simulink model "IEEE14_case"  (R2024b)
settings: Solver=FixedStepAuto  StartTime=0  StopTime=2  FixedStep=1e-7  RelTol=1e-3
values from neighbouring files (symbols this model uses):
  GFL_15_Bva = 0.009    [IEEE14_parameters.m]
  GFL_15_C_bus_pu = 7.179419    [IEEE14_parameters.m]
  GFL_15_f0 = 60    [IEEE14_parameters.m]
  GFL_15_I_id = 691.26967    [IEEE14_parameters.m]
  GFL_15_I_iq = 691.26967    [IEEE14_parameters.m]
  GFL_15_I_od = 45.2207    [IEEE14_parameters.m]
  GFL_15_I_oq = 45.2207    [IEEE14_parameters.m]
  GFL_15_I_pll = 0.78    [IEEE14_parameters.m]
  GFL_15_Kdi = 0.09    [IEEE14_parameters.m]
  GFL_15_Kdo = 0.9    [IEEE14_parameters.m]
  GFL_15_Kqi = 0.09    [IEEE14_parameters.m]
  GFL_15_Kqo = 0.9    [IEEE14_parameters.m]
  GFL_15_Lg_pu = 0.631447    [IEEE14_parameters.m]
  GFL_15_mode = 1    [IEEE14_parameters.m]
  GFL_15_P_id = 3.7166    [IEEE14_parameters.m]
  GFL_15_P_iq = 3.7166    [IEEE14_parameters.m]
  GFL_15_P_od = 0.4798    [IEEE14_parameters.m]
  GFL_15_P_oq = 0.4798    [IEEE14_parameters.m]
  GFL_15_P_pll = 290.42    [IEEE14_parameters.m]
  GFL_15_Qe_ref = 0.2    [IEEE14_parameters.m]
  GFL_15_Rg_pu = 0.024016    [IEEE14_parameters.m]
  GFL_15_Sbase = 1.000000e+4    (= 10000)    [IEEE14_parameters.m]
  GFL_15_Tdi = 0.01    [IEEE14_parameters.m]
  GFL_15_Tdo = 0.2    [IEEE14_parameters.m]
  GFL_15_Tqi = 0.01    [IEEE14_parameters.m]
  GFL_15_Tqo = 0.2    [IEEE14_parameters.m]
  GFL_15_Vbase = 380    [IEEE14_parameters.m]
  GFL_15_Vdc_ref = 1.011475    [IEEE14_parameters.m]
  GFL_15_Vdcbase = 700    [IEEE14_parameters.m]
  GFL_15_vq_ref = 0    [IEEE14_parameters.m]
  GFL_16_Bva = 0.002    [IEEE14_parameters.m]
  GFL_16_C_bus_pu = 7.179419    [IEEE14_parameters.m]
  GFL_16_f0 = 60    [IEEE14_parameters.m]
  GFL_16_I_id = 691.26967    [IEEE14_parameters.m]
  GFL_16_I_iq = 691.26967    [IEEE14_parameters.m]
  GFL_16_I_od = 45.2207    [IEEE14_parameters.m]
  GFL_16_I_oq = 45.2207    [IEEE14_parameters.m]
  GFL_16_I_pll = 0.78    [IEEE14_parameters.m]
  GFL_16_Kdi = 0.05    [IEEE14_parameters.m]
  GFL_16_Kdo = 0.5    [IEEE14_parameters.m]
  GFL_16_Kqi = 0.05    [IEEE14_parameters.m]
  GFL_16_Kqo = 0.5    [IEEE14_parameters.m]
  GFL_16_Lg_pu = 0.631447    [IEEE14_parameters.m]
  GFL_16_mode = 1    [IEEE14_parameters.m]
  GFL_16_P_id = 3.7166    [IEEE14_parameters.m]
  GFL_16_P_iq = 3.7166    [IEEE14_parameters.m]
  GFL_16_P_od = 0.4798    [IEEE14_parameters.m]
  GFL_16_P_oq = 0.4798    [IEEE14_parameters.m]
  GFL_16_P_pll = 290.42    [IEEE14_parameters.m]
  GFL_16_Qe_ref = 0.2    [IEEE14_parameters.m]
  GFL_16_Rg_pu = 0.024016    [IEEE14_parameters.m]
  GFL_16_Sbase = 1.000000e+4    (= 10000)    [IEEE14_parameters.m]
  GFL_16_Tdi = 0.01    [IEEE14_parameters.m]
  GFL_16_Tdo = 0.2    [IEEE14_parameters.m]
  GFL_16_Tqi = 0.01    [IEEE14_parameters.m]
  GFL_16_Tqo = 0.2    [IEEE14_parameters.m]
  GFL_16_Vbase = 380    [IEEE14_parameters.m]
  GFL_16_Vdc_ref = 1.01144    [IEEE14_parameters.m]
  GFL_16_Vdcbase = 700    [IEEE14_parameters.m]
  GFL_16_vq_ref = 0    [IEEE14_parameters.m]
  GFL_17_Bva = 0.002    [IEEE14_parameters.m]
  GFL_17_C_bus_pu = 7.179419    [IEEE14_parameters.m]
  GFL_17_f0 = 60    [IEEE14_parameters.m]
  GFL_17_I_id = 691.26967    [IEEE14_parameters.m]
  GFL_17_I_iq = 691.26967    [IEEE14_parameters.m]
  GFL_17_I_od = 45.2207    [IEEE14_parameters.m]
  GFL_17_I_oq = 45.2207    [IEEE14_parameters.m]
  GFL_17_I_pll = 0.78    [IEEE14_parameters.m]
  GFL_17_Kdi = 0.05    [IEEE14_parameters.m]
  GFL_17_Kdo = 0.5    [IEEE14_parameters.m]
  GFL_17_Kqi = 0.05    [IEEE14_parameters.m]
  GFL_17_Kqo = 0.5    [IEEE14_parameters.m]
  GFL_17_Lg_pu = 0.631447    [IEEE14_parameters.m]
  GFL_17_mode = 1    [IEEE14_parameters.m]
  GFL_17_P_id = 3.7166    [IEEE14_parameters.m]
  GFL_17_P_iq = 3.7166    [IEEE14_parameters.m]
  GFL_17_P_od = 0.4798    [IEEE14_parameters.m]
  GFL_17_P_oq = 0.4798    [IEEE14_parameters.m]
  GFL_17_P_pll = 290.42    [IEEE14_parameters.m]
  GFL_17_Qe_ref = 0.2    [IEEE14_parameters.m]
  GFL_17_Rg_pu = 0.024016    [IEEE14_parameters.m]
  GFL_17_Sbase = 1.000000e+4    (= 10000)    [IEEE14_parameters.m]
  GFL_17_Tdi = 0.01    [IEEE14_parameters.m]
  GFL_17_Tdo = 0.2    [IEEE14_parameters.m]
  GFL_17_Tqi = 0.01    [IEEE14_parameters.m]
  GFL_17_Tqo = 0.2    [IEEE14_parameters.m]
  GFL_17_Vbase = 380    [IEEE14_parameters.m]
  GFL_17_Vdc_ref = 1.011632    [IEEE14_parameters.m]
  GFL_17_Vdcbase = 700    [IEEE14_parameters.m]
  GFL_17_vq_ref = 0    [IEEE14_parameters.m]
  GFL_18_Bva = 0.002    [IEEE14_parameters.m]
  GFL_18_C_bus_pu = 7.179419    [IEEE14_parameters.m]
  GFL_18_f0 = 60    [IEEE14_parameters.m]
  GFL_18_I_id = 691.26967    [IEEE14_parameters.m]
  GFL_18_I_iq = 691.26967    [IEEE14_parameters.m]
  GFL_18_I_od = 45.2207    [IEEE14_parameters.m]
  GFL_18_I_oq = 45.2207    [IEEE14_parameters.m]
  GFL_18_I_pll = 0.78    [IEEE14_parameters.m]
  GFL_18_Kdi = 0.05    [IEEE14_parameters.m]
  GFL_18_Kdo = 0.5    [IEEE14_parameters.m]
  GFL_18_Kqi = 0.05    [IEEE14_parameters.m]
  GFL_18_Kqo = 0.5    [IEEE14_parameters.m]
  GFL_18_Lg_pu = 0.631447    [IEEE14_parameters.m]
  GFL_18_mode = 1    [IEEE14_parameters.m]
  GFL_18_P_id = 3.7166    [IEEE14_parameters.m]
  GFL_18_P_iq = 3.7166    [IEEE14_parameters.m]
  GFL_18_P_od = 0.4798    [IEEE14_parameters.m]
  GFL_18_P_oq = 0.4798    [IEEE14_parameters.m]
  GFL_18_P_pll = 290.42    [IEEE14_parameters.m]
  GFL_18_Qe_ref = 0.2    [IEEE14_parameters.m]
  GFL_18_Rg_pu = 0.024016    [IEEE14_parameters.m]
  GFL_18_Sbase = 1.000000e+4    (= 10000)    [IEEE14_parameters.m]
  GFL_18_Tdi = 0.01    [IEEE14_parameters.m]
  GFL_18_Tdo = 0.2    [IEEE14_parameters.m]
  GFL_18_Tqi = 0.01    [IEEE14_parameters.m]
  GFL_18_Tqo = 0.2    [IEEE14_parameters.m]
  GFL_18_Vbase = 380    [IEEE14_parameters.m]
  GFL_18_Vdc_ref = 1.011572    [IEEE14_parameters.m]
  GFL_18_Vdcbase = 700    [IEEE14_parameters.m]
  GFL_18_vq_ref = 0    [IEEE14_parameters.m]
  ... (+180 more)
(part 23 of 25)

== system IEEE14_case/SG_D_6/i_q_SG_D_6_block ==
  note: i_q_SG_D_6 in case14gfl
      | $-\frac{\sin\left(\theta _{\mathrm{SG},D,6}\right)\,\left(\psi _{q,\mathrm{SG},D,6}+\frac{\psi _{\mathrm{gq},\mathrm{SG},D,6}\,\left(x_{l}-x_{\mathrm{qdd}}\right)}{x_{l}-x_{\mathrm{qd}}}+\frac{\psi _{\mathrm{kq},\mathrm{SG},D,6}\,\left(x_{\mathrm{qd}}-x_{\mathrm{qdd}}\right)}{x_{l}-x_{\mathrm{qd}}}\right)}{x_{\mathrm{qdd}}}-\frac{\cos\left(\theta _{\mathrm{SG},D,6}\right)\,\left(\frac{\psi _{\mathrm{1d},\mathrm{SG},D,6}\,\left(x_{\mathrm{dd}}-x_{\mathrm{ddd}}\right)}{x_{\mathrm{dd}}-x_{l}}-\psi _{d,\mathrm{SG},D,6}+\frac{\psi _{\mathrm{fd},\mathrm{SG},D,6}\,\left(x_{\mathrm{ddd}}-x_{l}\right)}{x_{\mathrm{dd}}-x_{l}}\right)}{x_{\mathrm{ddd}}}$
      | Automatically generated on 2025-10-09 21:33:36 .
  State_psi_gq_SG_D_6_bb7cb : Inport
  State_psi_kq_SG_D_6_74fba : Inport  Port=2
  State_psi_q_SG_D_6_d539d : Inport  Port=3
  State_theta_SG_D_6_0f9f7 : Inport  Port=4
  State_psi_1d_SG_D_6_399cf : Inport  Port=5
  State_psi_d_SG_D_6_c39a1 : Inport  Port=6
  State_psi_fd_SG_D_6_27308 : Inport  Port=7
  State_theta_SG_D_6_711a7 : Inport  Port=8
  Add_1b784 : Sum
  Add_2059a : Sum
  Add_4e81d : Sum
  Add_a606b : Sum
  Add_b7e99 : Sum
  Add_bf051 : Sum
  Constant_-1_03d9f : Constant  Value=-1
  Constant_-1_3bc5f : Constant  Value=-1
  Constant_-1_c953a : Constant  Value=-1
  Constant_-1_fa54d : Constant  Value=-1
  Constant_-1_fd151 : Constant  Value=-1
  Constant_x_dd_00bb1 : Constant  Value=x_dd
  Constant_x_dd_b034c : Constant  Value=x_dd
  Constant_x_dd_da974 : Constant  Value=x_dd
  Constant_x_ddd_0990c : Constant  Value=x_ddd
  Constant_x_ddd_5aeff : Constant  Value=x_ddd
  Constant_x_ddd_89a1e : Constant  Value=x_ddd
  Constant_x_l_35cdf : Constant  Value=x_l
  Constant_x_l_39284 : Constant  Value=x_l
  Constant_x_l_426d4 : Constant  Value=x_l
  Constant_x_l_acd9f : Constant  Value=x_l
  Constant_x_l_d201c : Constant  Value=x_l
  Constant_x_l_e1d2c : Constant  Value=x_l
  Constant_x_qd_0187f : Constant  Value=x_qd
  Constant_x_qd_181c5 : Constant  Value=x_qd
  Constant_x_qd_da5c0 : Constant  Value=x_qd
  Constant_x_qdd_0b8ce : Constant  Value=x_qdd
  Constant_x_qdd_a7998 : Constant  Value=x_qdd
  Constant_x_qdd_d293e : Constant  Value=x_qdd
  Divide_1f5d5 : Product  Inputs=*/
  Divide_248c0 : Product  Inputs=*/
  Divide_5ce97 : Product  Inputs=*/
  Divide_aca68 : Product  Inputs=*/
  Divide_d3087 : Product  Inputs=*/
  Divide_df8a8 : Product  Inputs=*/
  MathFunc_cos_6c494 : Trigonometry  Operator=cos
  MathFunc_sin_3e9c3 : Trigonometry
  Product_1fff5 : Product
  Product_21479 : Product
  Product_2ea0e : Product
  Product_34123 : Product
  Product_6a3b1 : Product
  Product_74ee8 : Product
  Product_8b50b : Product
  Product_94998 : Product
  Product_ae5a3 : Product
  Product_b95d6 : Product
  Product_c3eb1 : Product
  Subtract_0660b : Sum  Inputs=+-
  Subtract_0dd9c : Sum  Inputs=+-
  Subtract_3e1a2 : Sum  Inputs=+-
  Subtract_4133d : Sum  Inputs=+-
  Subtract_b305f : Sum  Inputs=+-
  Subtract_ce2f2 : Sum  Inputs=+-
  Subtract_df7d1 : Sum  Inputs=+-
  Blockout_i_q_SG_D_6_da8c6 : Outport
  wires:
  Constant_x_dd_b034c/1 -> Subtract_ce2f2/1
  Constant_-1_fd151/1 -> Product_34123/1
  Constant_-1_fa54d/1 -> Product_2ea0e/1
  Subtract_4133d/1 -> Product_8b50b/2
  Constant_x_l_39284/1 -> Product_2ea0e/2
  Product_2ea0e/1 -> Add_bf051/1
  Constant_x_l_426d4/1 -> Subtract_0dd9c/2
  Constant_x_qdd_0b8ce/1 -> Subtract_df7d1/2
  Constant_x_qdd_d293e/1 -> Add_bf051/2
  Subtract_0dd9c/1 -> Product_1fff5/2
  Constant_x_qd_181c5/1 -> Subtract_df7d1/1
  Constant_x_l_35cdf/1 -> Subtract_ce2f2/2
  Add_bf051/1 -> Product_b95d6/2
  Constant_x_l_e1d2c/1 -> Product_34123/2
  Constant_-1_03d9f/1 -> Product_74ee8/1
  Constant_-1_c953a/1 -> Product_c3eb1/1
  Constant_x_l_acd9f/1 -> Product_74ee8/2
  State_theta_SG_D_6_0f9f7/1 -> MathFunc_sin_3e9c3/1
  State_psi_gq_SG_D_6_bb7cb/1 -> Product_b95d6/1
  Subtract_ce2f2/1 -> Divide_aca68/2
  Product_34123/1 -> Add_2059a/1
  State_psi_d_SG_D_6_c39a1/1 -> Add_1b784/2
  Constant_x_qd_0187f/1 -> Add_2059a/2
  Product_1fff5/1 -> Divide_1f5d5/1
  State_psi_kq_SG_D_6_74fba/1 -> Product_94998/1
  Subtract_df7d1/1 -> Product_94998/2
  Constant_x_dd_da974/1 -> Subtract_b305f/1
  Product_74ee8/1 -> Add_4e81d/1
  Constant_x_qd_da5c0/1 -> Add_4e81d/2
  State_psi_1d_SG_D_6_399cf/1 -> Product_c3eb1/2
  Constant_x_ddd_0990c/1 -> Divide_d3087/2
  Constant_x_dd_00bb1/1 -> Subtract_4133d/1
  MathFunc_sin_3e9c3/1 -> Product_21479/2
  Constant_x_ddd_89a1e/1 -> Subtract_4133d/2
  Add_b7e99/1 -> Product_ae5a3/2
  Product_b95d6/1 -> Divide_5ce97/1
  Add_2059a/1 -> Divide_5ce97/2
  Subtract_3e1a2/1 -> Add_b7e99/1
  Product_94998/1 -> Divide_248c0/1
  Add_4e81d/1 -> Divide_248c0/2
  Product_c3eb1/1 -> Product_8b50b/1
  Divide_df8a8/1 -> Add_a606b/1
  Constant_x_ddd_5aeff/1 -> Subtract_0dd9c/1
  Divide_5ce97/1 -> Subtract_3e1a2/1
  Divide_248c0/1 -> Subtract_3e1a2/2
  Product_8b50b/1 -> Divide_aca68/1
  State_psi_fd_SG_D_6_27308/1 -> Product_1fff5/1
  Constant_x_l_d201c/1 -> Subtract_b305f/2
  State_psi_q_SG_D_6_d539d/1 -> Add_b7e99/2
  Divide_aca68/1 -> Add_1b784/1
  Subtract_b305f/1 -> Divide_1f5d5/2
  Constant_-1_3bc5f/1 -> Product_ae5a3/1
  Add_1b784/1 -> Subtract_0660b/1
  Constant_x_qdd_a7998/1 -> Divide_df8a8/2
  Divide_1f5d5/1 -> Subtract_0660b/2
  State_theta_SG_D_6_711a7/1 -> MathFunc_cos_6c494/1
  Add_a606b/1 -> Blockout_i_q_SG_D_6_da8c6/1
  Product_ae5a3/1 -> Product_21479/1
  Subtract_0660b/1 -> Product_6a3b1/1
  MathFunc_cos_6c494/1 -> Product_6a3b1/2
  Divide_d3087/1 -> Add_a606b/2
  Product_21479/1 -> Divide_df8a8/1
  Product_6a3b1/1 -> Divide_d3087/1

== system IEEE14_case/SG_D_6/theta_SG_D_6_out_block ==
  note: theta_SG_D_6_out in case14gfl
      | $\theta _{\mathrm{SG},D,6}$
      | Automatically generated on 2025-10-09 21:33:41 .
  State_theta_SG_D_6_29a7d : Inport
  Blockout_theta_SG_D_6_out_e355f : Outport
  wires:
  State_theta_SG_D_6_29a7d/1 -> Blockout_theta_SG_D_6_out_e355f/1

== system IEEE14_case/SG_D_6/w_SG_D_6_out_block ==
  note: w_SG_D_6_out in case14gfl
      | $w_{\mathrm{SG},D,6}$
      | Automatically generated on 2025-10-09 21:33:41 .
  State_w_SG_D_6_51261 : Inport
  Blockout_w_SG_D_6_out_90215 : Outport
  wires:
  State_w_SG_D_6_51261/1 -> Blockout_w_SG_D_6_out_90215/1

== system IEEE14_case/SG_D_8/T_e_SG_D_8_block ==
  note: T_e_SG_D_8 in case14gfl
      | $-\frac{\psi _{d,\mathrm{SG},D,8}\,\left(\psi _{q,\mathrm{SG},D,8}+\frac{\psi _{\mathrm{gq},\mathrm{SG},D,8}\,\left(x_{l}-x_{\mathrm{qdd}}\right)}{x_{l}-x_{\mathrm{qd}}}+\frac{\psi _{\mathrm{kq},\mathrm{SG},D,8}\,\left(x_{\mathrm{qd}}-x_{\mathrm{qdd}}\right)}{x_{l}-x_{\mathrm{qd}}}\right)}{x_{\mathrm{qdd}}}-\frac{\psi _{q,\mathrm{SG},D,8}\,\left(\frac{\psi _{\mathrm{1d},\mathrm{SG},D,8}\,\left(x_{\mathrm{dd}}-x_{\mathrm{ddd}}\right)}{x_{\mathrm{dd}}-x_{l}}-\psi _{d,\mathrm{SG},D,8}+\frac{\psi _{\mathrm{fd},\mathrm{SG},D,8}\,\left(x_{\mathrm{ddd}}-x_{l}\right)}{x_{\mathrm{dd}}-x_{l}}\right)}{x_{\mathrm{ddd}}}$
      | Automatically generated on 2025-10-09 21:34:39 .
  State_psi_d_SG_D_8_8bce2 : Inport
  State_psi_gq_SG_D_8_ece9e : Inport  Port=2
  State_psi_kq_SG_D_8_39808 : Inport  Port=3
  State_psi_q_SG_D_8_1c36c : Inport  Port=4
  State_psi_q_SG_D_8_67075 : Inport  Port=5
  State_psi_1d_SG_D_8_d92c8 : Inport  Port=6
  State_psi_d_SG_D_8_41989 : Inport  Port=7
  State_psi_fd_SG_D_8_0a0bc : Inport  Port=8
  Add_06b69 : Sum
  Add_59326 : Sum
  Add_632ff : Sum
  Add_c3923 : Sum
  Add_cadb4 : Sum
  Add_f94cb : Sum
  Constant_-1_2e741 : Constant  Value=-1
  Constant_-1_4359c : Constant  Value=-1
  Constant_-1_8aae0 : Constant  Value=-1
  Constant_-1_a07ac : Constant  Value=-1
  Constant_-1_d0e0d : Constant  Value=-1
  Constant_x_dd_3484e : Constant  Value=x_dd
  Constant_x_dd_60afc : Constant  Value=x_dd
  Constant_x_dd_f506f : Constant  Value=x_dd
  Constant_x_ddd_43954 : Constant  Value=x_ddd
  Constant_x_ddd_a007d : Constant  Value=x_ddd
  Constant_x_ddd_f20a3 : Constant  Value=x_ddd
  Constant_x_l_0e8b4 : Constant  Value=x_l
  Constant_x_l_69aef : Constant  Value=x_l
  Constant_x_l_d6c60 : Constant  Value=x_l
  Constant_x_l_d7c13 : Constant  Value=x_l
  Constant_x_l_f15ed : Constant  Value=x_l
  Constant_x_l_f66ab : Constant  Value=x_l
  Constant_x_qd_29c71 : Constant  Value=x_qd
  Constant_x_qd_3b3c5 : Constant  Value=x_qd
  Constant_x_qd_aaedd : Constant  Value=x_qd
  Constant_x_qdd_6fb08 : Constant  Value=x_qdd
  Constant_x_qdd_cc47d : Constant  Value=x_qdd
  Constant_x_qdd_f6893 : Constant  Value=x_qdd
  Divide_46739 : Product  Inputs=*/
  Divide_5b4a1 : Product  Inputs=*/
  Divide_7591d : Product  Inputs=*/
  Divide_9ac0b : Product  Inputs=*/
  Divide_daa4b : Product  Inputs=*/
  Divide_e15ac : Product  Inputs=*/
  Product_1ea96 : Product
  Product_3e5e0 : Product
  Product_46d7e : Product
  Product_6dfe9 : Product
  Product_a7ae5 : Product
  Product_ad0f4 : Product
  Product_ae9a5 : Product
  Product_c7dff : Product
  Product_ce19d : Product
  Product_d5235 : Product
  Product_f69c7 : Product
  Subtract_4614f : Sum  Inputs=+-
  Subtract_8bdef : Sum  Inputs=+-
  Subtract_9a288 : Sum  Inputs=+-
  Subtract_a8a93 : Sum  Inputs=+-
  Subtract_cfacb : Sum  Inputs=+-
  Subtract_e2590 : Sum  Inputs=+-
  Subtract_f13c7 : Sum  Inputs=+-
  Blockout_T_e_SG_D_8_36eef : Outport
  wires:
  Product_ce19d/1 -> Divide_5b4a1/1
  Constant_-1_4359c/1 -> Product_1ea96/1
  Constant_x_l_69aef/1 -> Product_1ea96/2
  Add_06b69/1 -> Subtract_a8a93/1
  State_psi_fd_SG_D_8_0a0bc/1 -> Product_3e5e0/1
  Constant_x_qdd_f6893/1 -> Add_59326/2
  Constant_x_qdd_cc47d/1 -> Subtract_8bdef/2
  Add_cadb4/1 -> Product_ae9a5/2
  Product_1ea96/1 -> Add_59326/1
  Constant_-1_8aae0/1 -> Product_46d7e/1
  Product_c7dff/1 -> Add_632ff/1
  Constant_x_l_0e8b4/1 -> Product_46d7e/2
  State_psi_d_SG_D_8_41989/1 -> Add_06b69/2
  Constant_x_qd_29c71/1 -> Subtract_8bdef/1
  Constant_x_qd_3b3c5/1 -> Add_c3923/2
  Constant_-1_a07ac/1 -> Product_c7dff/1
  Subtract_9a288/1 -> Divide_daa4b/2
  Constant_x_l_f66ab/1 -> Product_c7dff/2
  Product_6dfe9/1 -> Product_ad0f4/1
  Constant_-1_d0e0d/1 -> Product_6dfe9/1
  Divide_5b4a1/1 -> Subtract_4614f/2
  State_psi_1d_SG_D_8_d92c8/1 -> Product_6dfe9/2
  Product_d5235/1 -> Product_ae9a5/1
  Divide_9ac0b/1 -> Add_06b69/1
  Subtract_f13c7/1 -> Product_ad0f4/2
  Constant_x_dd_60afc/1 -> Subtract_f13c7/1
  Constant_x_ddd_f20a3/1 -> Subtract_f13c7/2
  State_psi_gq_SG_D_8_ece9e/1 -> Product_a7ae5/1
  Add_59326/1 -> Product_a7ae5/2
  Divide_daa4b/1 -> Subtract_a8a93/2
  Product_46d7e/1 -> Add_c3923/1
  Product_a7ae5/1 -> Divide_46739/1
  State_psi_kq_SG_D_8_39808/1 -> Product_ce19d/1
  Subtract_8bdef/1 -> Product_ce19d/2
  Add_c3923/1 -> Divide_46739/2
  Constant_x_qd_aaedd/1 -> Add_632ff/2
  Subtract_e2590/1 -> Divide_9ac0b/2
  Constant_x_dd_3484e/1 -> Subtract_e2590/1
  State_psi_q_SG_D_8_1c36c/1 -> Add_cadb4/2
  Subtract_4614f/1 -> Add_cadb4/1
  Constant_x_l_f15ed/1 -> Subtract_e2590/2
  Constant_x_ddd_43954/1 -> Subtract_cfacb/1
  Constant_x_l_d7c13/1 -> Subtract_cfacb/2
  Add_632ff/1 -> Divide_5b4a1/2
  Product_ad0f4/1 -> Divide_9ac0b/1
  Divide_46739/1 -> Subtract_4614f/1
  Subtract_cfacb/1 -> Product_3e5e0/2
  Constant_x_dd_f506f/1 -> Subtract_9a288/1
  Constant_x_l_d6c60/1 -> Subtract_9a288/2
  State_psi_d_SG_D_8_8bce2/1 -> Product_d5235/2
  Product_3e5e0/1 -> Divide_daa4b/1
  Constant_-1_2e741/1 -> Product_d5235/1
  Product_f69c7/1 -> Divide_7591d/1
  State_psi_q_SG_D_8_67075/1 -> Product_f69c7/1
  Subtract_a8a93/1 -> Product_f69c7/2
  Product_ae9a5/1 -> Divide_e15ac/1
  Constant_x_qdd_6fb08/1 -> Divide_e15ac/2
  Constant_x_ddd_a007d/1 -> Divide_7591d/2
  Divide_e15ac/1 -> Add_f94cb/1
  Divide_7591d/1 -> Add_f94cb/2
  Add_f94cb/1 -> Blockout_T_e_SG_D_8_36eef/1

== system IEEE14_case/SG_D_8/d_E_fd_SG_D_8_block ==
  note: d_E_fd_SG_D_8 in case14gfl
      | $\frac{V_{f,\mathrm{SG},D,8}-E_{\mathrm{fd},\mathrm{SG},D,8}\,K_{E}}{T_{E}}$
      | Automatically generated on 2025-10-09 21:34:26 .
  State_E_fd_SG_D_8_6df86 : Inport
  State_V_f_SG_D_8_2f3e7 : Inport  Port=2
  Add_66a63 : Sum
  Constant_-1_ef80b : Constant  Value=-1
  Constant_K_E_8957f : Constant  Value=K_E
  Constant_T_E_afa68 : Constant  Value=T_E
  Divide_746d8 : Product  Inputs=*/
  Product_bbc24 : Product
  Product_e8239 : Product
  Blockout_d_E_fd_SG_D_8_bd076 : Outport
  wires:
  State_V_f_SG_D_8_2f3e7/1 -> Add_66a63/2
  State_E_fd_SG_D_8_6df86/1 -> Product_e8239/2
  Constant_-1_ef80b/1 -> Product_e8239/1
  Constant_T_E_afa68/1 -> Divide_746d8/2
  Product_e8239/1 -> Product_bbc24/1
  Constant_K_E_8957f/1 -> Product_bbc24/2
  Add_66a63/1 -> Divide_746d8/1
  Divide_746d8/1 -> Blockout_d_E_fd_SG_D_8_bd076/1
  Product_bbc24/1 -> Add_66a63/1

== system IEEE14_case/SG_D_8/d_Px_1_SG_D_8_block ==
  note: d_Px_1_SG_D_8 in case14gfl
      | $\frac{w_{\mathrm{SG},D,8}-2\,\pi \,f_{0}}{T_{w}}-\frac{\mathrm{Px}_{1,\mathrm{SG},D,8}}{T_{w}}$
      | Automatically generated on 2025-10-09 21:34:27 .
  State_Px_1_SG_D_8_6e138 : Inport
  State_w_SG_D_8_14513 : Inport  Port=2
  Add_6e344 : Sum
  Add_c31f2 : Sum
  Constant_-1_ef042 : Constant  Value=-1
  Constant_-2.0_f57a6 : Constant  Value=-2.0
  Constant_T_w_34630 : Constant  Value=T_w
  Constant_T_w_4eda6 : Constant  Value=T_w
  Constant_f0_4a4a4 : Constant  Value=f0
  Constant_pi_a2580 : Constant  Value=pi
  Divide_32cd3 : Product  Inputs=*/
  Divide_7bde2 : Product  Inputs=*/
  Product_6840a : Product
  Product_89240 : Product
  Product_dbed8 : Product
  Blockout_d_Px_1_SG_D_8_010b5 : Outport
  wires:
  Constant_-2.0_f57a6/1 -> Product_6840a/1
  Product_6840a/1 -> Product_dbed8/1
  Constant_-1_ef042/1 -> Product_89240/1
  Constant_pi_a2580/1 -> Product_6840a/2
  Constant_f0_4a4a4/1 -> Product_dbed8/2
  State_Px_1_SG_D_8_6e138/1 -> Product_89240/2
  Add_6e344/1 -> Divide_32cd3/1
  Product_89240/1 -> Divide_7bde2/1
  Product_dbed8/1 -> Add_6e344/1
  State_w_SG_D_8_14513/1 -> Add_6e344/2
  Constant_T_w_4eda6/1 -> Divide_7bde2/2
  Constant_T_w_34630/1 -> Divide_32cd3/2
  Divide_7bde2/1 -> Add_c31f2/1
  Divide_32cd3/1 -> Add_c31f2/2
  Add_c31f2/1 -> Blockout_d_Px_1_SG_D_8_010b5/1

== system IEEE14_case/SG_D_8/d_Px_2_SG_D_8_block ==
  note: d_Px_2_SG_D_8 in case14gfl
      | $\frac{\mathrm{Px}_{1,\mathrm{SG},D,8}-T_{2}\,\left(\frac{\mathrm{Px}_{1,\mathrm{SG},D,8}}{T_{w}}-\frac{w_{\mathrm{SG},D,8}-2\,\pi \,f_{0}}{T_{w}}\right)}{T_{1}}-\frac{\mathrm{Px}_{2,\mathrm{SG},D,8}}{T_{1}}$
      | Automatically generated on 2025-10-09 21:34:28 .
  State_Px_2_SG_D_8_4dc99 : Inport
  State_Px_1_SG_D_8_d499c : Inport  Port=2
  State_Px_1_SG_D_8_35ac2 : Inport  Port=3
  State_w_SG_D_8_213d1 : Inport  Port=4
  Add_02c0f : Sum
  Add_3c4c5 : Sum
  Add_c9069 : Sum
  Add_f1b35 : Sum
  Constant_-1_dce63 : Constant  Value=-1
  Constant_-1_f1a3f : Constant  Value=-1
  Constant_-2.0_19730 : Constant  Value=-2.0
  Constant_T_1_8c6d2 : Constant  Value=T_1
  Constant_T_1_8f1dd : Constant  Value=T_1
  Constant_T_2_97cff : Constant  Value=T_2
  Constant_T_w_50747 : Constant  Value=T_w
  Constant_T_w_78d3a : Constant  Value=T_w
  Constant_f0_22743 : Constant  Value=f0
  Constant_pi_f77ee : Constant  Value=pi
  Divide_94fbb : Product  Inputs=*/
  Divide_c0a4f : Product  Inputs=*/
  Divide_f4425 : Product  Inputs=*/
  Divide_ffc10 : Product  Inputs=*/
  Product_14280 : Product
  Product_288d1 : Product
  Product_3bc5b : Product
  Product_4555b : Product
  Product_93d10 : Product
  Blockout_d_Px_2_SG_D_8_ad385 : Outport
  wires:
  Constant_-2.0_19730/1 -> Product_93d10/1
  Constant_pi_f77ee/1 -> Product_93d10/2
  Product_93d10/1 -> Product_3bc5b/1
  State_Px_1_SG_D_8_35ac2/1 -> Product_288d1/2
  Constant_f0_22743/1 -> Product_3bc5b/2
  State_w_SG_D_8_213d1/1 -> Add_02c0f/2
  Constant_-1_dce63/1 -> Product_288d1/1
  Constant_T_1_8c6d2/1 -> Divide_ffc10/2
  Product_3bc5b/1 -> Add_02c0f/1
  Product_288d1/1 -> Divide_94fbb/1
  Constant_T_w_78d3a/1 -> Divide_94fbb/2
  State_Px_2_SG_D_8_4dc99/1 -> Product_4555b/2
  Add_02c0f/1 -> Divide_f4425/1
  Constant_T_w_50747/1 -> Divide_f4425/2
  Divide_94fbb/1 -> Add_3c4c5/1
  Divide_f4425/1 -> Add_3c4c5/2
  Product_14280/1 -> Add_c9069/2
  Constant_T_2_97cff/1 -> Product_14280/1
  Add_3c4c5/1 -> Product_14280/2
  Constant_-1_f1a3f/1 -> Product_4555b/1
  Add_c9069/1 -> Divide_c0a4f/1
  Product_4555b/1 -> Divide_ffc10/1
  State_Px_1_SG_D_8_d499c/1 -> Add_c9069/1
  Constant_T_1_8f1dd/1 -> Divide_c0a4f/2
  Divide_ffc10/1 -> Add_f1b35/1
  Divide_c0a4f/1 -> Add_f1b35/2
  Add_f1b35/1 -> Blockout_d_Px_2_SG_D_8_ad385/1

== system IEEE14_case/SG_D_8/d_Px_3_SG_D_8_block ==
  note: d_Px_3_SG_D_8 in case14gfl
      | $\frac{\mathrm{Px}_{2,\mathrm{SG},D,8}+T_{4}\,\left(\frac{\mathrm{Px}_{1,\mathrm{SG},D,8}-T_{2}\,\left(\frac{\mathrm{Px}_{1,\mathrm{SG},D,8}}{T_{w}}-\frac{w_{\mathrm{SG},D,8}-2\,\pi \,f_{0}}{T_{w}}\right)}{T_{1}}-\frac{\mathrm{Px}_{2,\mathrm{SG},D,8}}{T_{1}}\right)}{T_{3}}-\frac{\mathrm{Px}_{3,\mathrm{SG},D,8}}{T_{3}}$
      | Automatically generated on 2025-10-09 21:34:30 .
  State_Px_3_SG_D_8_df285 : Inport
  State_Px_2_SG_D_8_f1029 : Inport  Port=2
  State_Px_2_SG_D_8_bb5ac : Inport  Port=3
  State_Px_1_SG_D_8_7f9bd : Inport  Port=4
  State_Px_1_SG_D_8_8b47e : Inport  Port=5
  State_w_SG_D_8_deb3f : Inport  Port=6
  Add_5fe36 : Sum
  Add_6979a : Sum
  Add_6d7ab : Sum
  Add_819d5 : Sum
  Add_90b30 : Sum
  Add_e384d : Sum
  Constant_-1_35062 : Constant  Value=-1
  Constant_-1_66af6 : Constant  Value=-1
  Constant_-1_d88cf : Constant  Value=-1
  Constant_-2.0_56047 : Constant  Value=-2.0
  Constant_T_1_9cf83 : Constant  Value=T_1
  Constant_T_1_d8cdf : Constant  Value=T_1
  Constant_T_2_e57ea : Constant  Value=T_2
  Constant_T_3_5c7ed : Constant  Value=T_3
  Constant_T_3_fb0f8 : Constant  Value=T_3
  Constant_T_4_6ad58 : Constant  Value=T_4
  Constant_T_w_86336 : Constant  Value=T_w
  Constant_T_w_fba3d : Constant  Value=T_w
  Constant_f0_1ed8a : Constant  Value=f0
  Constant_pi_2aa6c : Constant  Value=pi
  Divide_03bb6 : Product  Inputs=*/
  Divide_18d06 : Product  Inputs=*/
  Divide_2db84 : Product  Inputs=*/
  Divide_a5bfd : Product  Inputs=*/
  Divide_a8711 : Product  Inputs=*/
  Divide_e5bf0 : Product  Inputs=*/
  Product_1ae8e : Product
  Product_26b25 : Product
  Product_5d23e : Product
  Product_61971 : Product
  Product_6cc1b : Product
  Product_76fa5 : Product
  Product_cbc0f : Product
  Blockout_d_Px_3_SG_D_8_b7d57 : Outport
  wires:
  Constant_-2.0_56047/1 -> Product_76fa5/1
  Constant_pi_2aa6c/1 -> Product_76fa5/2
  State_Px_3_SG_D_8_df285/1 -> Product_61971/2
  Product_76fa5/1 -> Product_cbc0f/1
  State_Px_1_SG_D_8_8b47e/1 -> Product_5d23e/2
  Constant_f0_1ed8a/1 -> Product_cbc0f/2
  State_w_SG_D_8_deb3f/1 -> Add_e384d/2
  Constant_-1_d88cf/1 -> Product_5d23e/1
  Product_cbc0f/1 -> Add_e384d/1
  Divide_18d06/1 -> Add_6979a/1
  Product_5d23e/1 -> Divide_e5bf0/1
  Constant_T_w_86336/1 -> Divide_e5bf0/2
  Add_e384d/1 -> Divide_2db84/1
  Constant_T_w_fba3d/1 -> Divide_2db84/2
  Divide_e5bf0/1 -> Add_5fe36/1
  Divide_2db84/1 -> Add_5fe36/2
  Divide_a8711/1 -> Add_6979a/2
  Constant_-1_35062/1 -> Product_61971/1
  Product_1ae8e/1 -> Add_6d7ab/2
  Constant_T_2_e57ea/1 -> Product_1ae8e/1
  Add_5fe36/1 -> Product_1ae8e/2
  Product_6cc1b/1 -> Divide_03bb6/1
  Constant_-1_66af6/1 -> Product_6cc1b/1
  State_Px_2_SG_D_8_bb5ac/1 -> Product_6cc1b/2
  Add_6d7ab/1 -> Divide_a5bfd/1
  State_Px_1_SG_D_8_7f9bd/1 -> Add_6d7ab/1
  Constant_T_1_d8cdf/1 -> Divide_03bb6/2
  Constant_T_1_9cf83/1 -> Divide_a5bfd/2
  Divide_03bb6/1 -> Add_90b30/1
  Divide_a5bfd/1 -> Add_90b30/2
  Product_26b25/1 -> Add_819d5/2
  Constant_T_4_6ad58/1 -> Product_26b25/1
  Add_90b30/1 -> Product_26b25/2
  Add_819d5/1 -> Divide_a8711/1
  State_Px_2_SG_D_8_f1029/1 -> Add_819d5/1
  Product_61971/1 -> Divide_18d06/1
  Constant_T_3_5c7ed/1 -> Divide_a8711/2
  Constant_T_3_fb0f8/1 -> Divide_18d06/2
  Add_6979a/1 -> Blockout_d_Px_3_SG_D_8_b7d57/1

== system IEEE14_case/SG_D_8/d_R_f_SG_D_8_block ==
  note: d_R_f_SG_D_8 in case14gfl
      | $-\frac{R_{f,\mathrm{SG},D,8}-\frac{E_{\mathrm{fd},\mathrm{SG},D,8}\,K_{F}}{T_{F}}}{T_{F}}$
      | Automatically generated on 2025-10-09 21:34:25 .
  State_E_fd_SG_D_8_d418e : Inport
  State_R_f_SG_D_8_19ab3 : Inport  Port=2
  Constant_K_F_d5c0f : Constant  Value=K_F
  Constant_T_F_983c8 : Constant  Value=T_F
  Constant_T_F_afa44 : Constant  Value=T_F
  Divide_4f781 : Product  Inputs=*/
  Divide_f89fb : Product  Inputs=*/
  Product_ec40c : Product
  Subtract_32c5f : Sum  Inputs=+-
  Blockout_d_R_f_SG_D_8_431b8 : Outport
  wires:
  State_E_fd_SG_D_8_d418e/1 -> Product_ec40c/1
  Divide_4f781/1 -> Subtract_32c5f/1
  Constant_K_F_d5c0f/1 -> Product_ec40c/2
  Product_ec40c/1 -> Divide_4f781/1
  Constant_T_F_983c8/1 -> Divide_4f781/2
  State_R_f_SG_D_8_19ab3/1 -> Subtract_32c5f/2
  Constant_T_F_afa44/1 -> Divide_f89fb/2
  Subtract_32c5f/1 -> Divide_f89fb/1
  Divide_f89fb/1 -> Blockout_d_R_f_SG_D_8_431b8/1

== system IEEE14_case/SG_D_8/d_T_m_SG_D_8_block ==
  note: d_T_m_SG_D_8 in case14gfl
      | $-\frac{T_{m,\mathrm{SG},D,8}-T_{0}+\frac{\mathrm{SpeedPara}\,\left(w_{\mathrm{SG},D,8}-w_{\mathrm{ref}}\right)}{2\,f_{0}\,\pi }}{T_{\mathrm{speed}}}$
      | Automatically generated on 2025-10-09 21:34:17 .
  State_w_SG_D_8_04413 : Inport
  State_T_m_SG_D_8_6d384 : Inport  Port=2
  Add_39575 : Sum
  Add_658eb : Sum
  Constant_-1_71780 : Constant  Value=-1
  Constant_2.0_c29ec : Constant  Value=2.0
  Constant_SpeedPara_b1470 : Constant  Value=SpeedPara
  Constant_T_0_7a148 : Constant  Value=T_0
  Constant_T_speed_8e42e : Constant  Value=T_speed
  Constant_f0_42534 : Constant  Value=f0
  Constant_pi_d582c : Constant  Value=pi
  Constant_w_ref_509bf : Constant  Value=w_ref
  Divide_547b3 : Product  Inputs=*/
  Divide_c135c : Product  Inputs=*/
  Product_14f8b : Product
  Product_6a631 : Product
  Product_9694e : Product
  Product_c38ae : Product
  Subtract_bcc29 : Sum  Inputs=+-
  Blockout_d_T_m_SG_D_8_65767 : Outport
  wires:
  Constant_SpeedPara_b1470/1 -> Product_14f8b/1
  State_w_SG_D_8_04413/1 -> Product_c38ae/2
  Constant_-1_71780/1 -> Product_c38ae/1
  Constant_2.0_c29ec/1 -> Product_9694e/1
  Product_c38ae/1 -> Add_39575/1
  Constant_T_0_7a148/1 -> Add_658eb/2
  Constant_w_ref_509bf/1 -> Add_39575/2
  Add_39575/1 -> Product_14f8b/2
  Constant_pi_d582c/1 -> Product_9694e/2
  Product_9694e/1 -> Product_6a631/1
  Constant_f0_42534/1 -> Product_6a631/2
  Product_14f8b/1 -> Divide_547b3/1
  Product_6a631/1 -> Divide_547b3/2
  Divide_547b3/1 -> Add_658eb/1
  Add_658eb/1 -> Subtract_bcc29/1
  State_T_m_SG_D_8_6d384/1 -> Subtract_bcc29/2
  Subtract_bcc29/1 -> Divide_c135c/1
  Constant_T_speed_8e42e/1 -> Divide_c135c/2
  Divide_c135c/1 -> Blockout_d_T_m_SG_D_8_65767/1

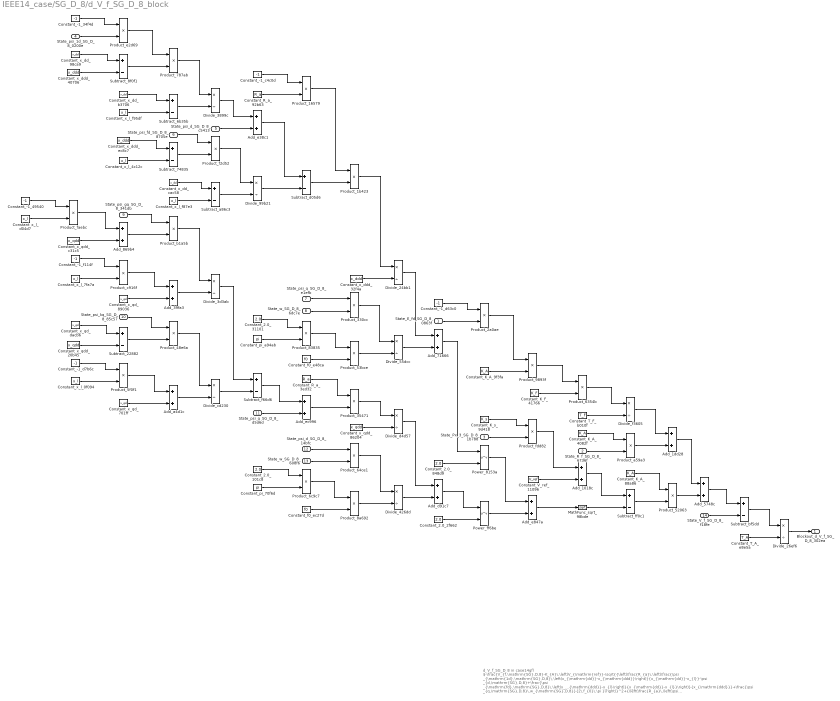
== system IEEE14_case/SG_D_8/d_V_f_SG_D_8_block ==
  note: d_V_f_SG_D_8 in case14gfl
      | $-\frac{V_{f,\mathrm{SG},D,8}-K_{A}\,\left(V_{\mathrm{ref}}-\sqrt{{\left(\frac{R_{a}\,\left(\frac{\psi _{\mathrm{1d},\mathrm{SG},D,8}\,\left(x_{\mathrm{dd}}-x_{\mathrm{ddd}}\right)}{x_{\mathrm{dd}}-x_{l}}-\psi _{d,\mathrm{SG},D,8}+\frac{\psi _{\mathrm{fd},\mathrm{SG},D,8}\,\left(x_{\mathrm{ddd}}-x_{l}\right)}{x_{\mathrm{dd}}-x_{l}}\right)}{x_{\mathrm{ddd}}}+\frac{\psi _{q,\mathrm{SG},D,8}\,w_{\mathrm{SG},D,8}}{2\,f_{0}\,\pi }\right)}^2+{\left(\frac{R_{a}\,\left(\psi _{q,\mathrm{SG},D,8}+\frac{\psi _{\mathrm{gq},\mathrm{SG},D,8}\,\left(x_{l}-x_{\mathrm{qdd}}\right)}{x_{l}-x_{\mathrm{qd}}}+\frac{\psi _{\mathrm{kq},\mathrm{SG},D,8}\,\left(x_{\mathrm{qd}}-x_{\mathrm{qdd}}\right)}{x_{l}-x_{\mathrm{qd}}}\right)}{x_{\mathrm{qdd}}}+\frac{\psi _{d,\mathrm{SG},D,8}\,w_{\mathrm{SG},D,8}}{2\,f_{0}\,\pi }\right)}^2}+K_{s}\,\mathrm{Px}_{3,\mathrm{SG},D,8}\right)-K_{A}\,R_{f,\mathrm{SG},D,8}+\frac{E_{\mathrm{fd},\mathrm{SG},D,8}\,K_{A}\,K_{F}}{T_{F}}}{T_{A}}$
      | Automatically generated on 2025-10-09 21:34:23 .
  State_E_fd_SG_D_8_0863f : Inport
  State_R_f_SG_D_8_6736f : Inport  Port=2
  State_Px_3_SG_D_8_1b788 : Inport  Port=3
  State_psi_1d_SG_D_8_0200e : Inport  Port=4
  State_psi_d_SG_D_8_c5413 : Inport  Port=5
  State_psi_fd_SG_D_8_8705e : Inport  Port=6
  State_psi_q_SG_D_8_e1efb : Inport  Port=7
  State_w_SG_D_8_6dc7e : Inport  Port=8
  State_psi_gq_SG_D_8_341db : Inport  Port=9
  State_psi_kq_SG_D_8_85c57 : Inport  Port=10
  State_psi_q_SG_D_8_d5d6d : Inport  Port=11
  State_psi_d_SG_D_8_14bfc : Inport  Port=12
  State_w_SG_D_8_608f6 : Inport  Port=13
  State_V_f_SG_D_8_f18fe : Inport  Port=14
  Add_1018c : Sum
  Add_1dd28 : Sum
  Add_39fa3 : Sum
  Add_5748c : Sum
  Add_71666 : Sum
  Add_869b4 : Sum
  Add_a4d1c : Sum
  Add_d91c7 : Sum
  Add_e38c1 : Sum
  Add_e847a : Sum
  Add_ec996 : Sum
  Constant_-1_34f4d : Constant  Value=-1
  Constant_-1_49540 : Constant  Value=-1
  Constant_-1_c4c0d : Constant  Value=-1
  Constant_-1_d63c0 : Constant  Value=-1
  Constant_-1_d7b6c : Constant  Value=-1
  Constant_-1_f114f : Constant  Value=-1
  Constant_2.0_101c8 : Constant  Value=2.0
  Constant_2.0_2f662 : Constant  Value=2.0
  Constant_2.0_31101 : Constant  Value=2.0
  Constant_2.0_848d9 : Constant  Value=2.0
  Constant_K_A_4082f : Constant  Value=K_A
  Constant_K_A_88a86 : Constant  Value=K_A
  Constant_K_A_9f3fa : Constant  Value=K_A
  Constant_K_F_41766 : Constant  Value=K_F
  Constant_K_s_9d418 : Constant  Value=K_s
  Constant_R_a_3ed32 : Constant  Value=R_a
  Constant_R_a_92b63 : Constant  Value=R_a
  Constant_T_A_e8e5a : Constant  Value=T_A
  Constant_T_F_b010f : Constant  Value=T_F
  Constant_V_ref_11096 : Constant  Value=V_ref
  Constant_f0_e48ca : Constant  Value=f0
  Constant_f0_ec27d : Constant  Value=f0
  Constant_pi_70f6d : Constant  Value=pi
  Constant_pi_a94ab : Constant  Value=pi
  Constant_x_dd_98ca9 : Constant  Value=x_dd
  Constant_x_dd_b3706 : Constant  Value=x_dd
  Constant_x_dd_cac58 : Constant  Value=x_dd
  Constant_x_ddd_32f4a : Constant  Value=x_ddd
  Constant_x_ddd_40706 : Constant  Value=x_ddd
  Constant_x_ddd_ec8c7 : Constant  Value=x_ddd
  Constant_x_l_0f094 : Constant  Value=x_l
  Constant_x_l_4c12c : Constant  Value=x_l
  Constant_x_l_7fa7a : Constant  Value=x_l
  Constant_x_l_d04d7 : Constant  Value=x_l
  Constant_x_l_f87e3 : Constant  Value=x_l
  Constant_x_l_f95df : Constant  Value=x_l
  Constant_x_qd_701ff : Constant  Value=x_qd
  Constant_x_qd_89036 : Constant  Value=x_qd
  Constant_x_qd_dacb6 : Constant  Value=x_qd
  Constant_x_qdd_20b45 : Constant  Value=x_qdd
  Constant_x_qdd_86204 : Constant  Value=x_qdd
  Constant_x_qdd_c31c5 : Constant  Value=x_qdd
  Divide_24bb1 : Product  Inputs=*/
  Divide_26ef6 : Product  Inputs=*/
  Divide_3899c : Product  Inputs=*/
  Divide_3d3ab : Product  Inputs=*/
  Divide_426dd : Product  Inputs=*/
  Divide_55dcc : Product  Inputs=*/
  Divide_99b21 : Product  Inputs=*/
  Divide_cd230 : Product  Inputs=*/
  Divide_d4d57 : Product  Inputs=*/
  Divide_f3605 : Product  Inputs=*/
  MathFunc_sqrt_98bde : Sqrt
  Power_8153a : Math  Operator=pow
  Power_ff6be : Math  Operator=pow
  Product_{16579,35471,52063,83835} (4 alike) : Product
  Product_1b423 : Product
  Product_2a0ae : Product
  Product_330cc : Product
  Product_48e6a : Product
  Product_53bce : Product
  Product_5f0f1 : Product
  Product_6354b : Product
  Product_64ce1 : Product
  Product_6c9c7 : Product
  Product_787ab : Product
  Product_8a692 : Product
  Product_9893f : Product
  Product_a59a3 : Product
  Product_b1a5b : Product
  Product_c916f : Product
  Product_e2d69 : Product
  Product_f2d52 : Product
  Product_faebc : Product
  Product_fdd82 : Product
  Subtract_22882 : Sum  Inputs=+-
  Subtract_6b35b : Sum  Inputs=+-
  Subtract_74835 : Sum  Inputs=+-
  Subtract_8f0f1 : Sum  Inputs=+-
  Subtract_a86c3 : Sum  Inputs=+-
  Subtract_bf5dd : Sum  Inputs=+-
  Subtract_d05d6 : Sum  Inputs=+-
  Subtract_f66d6 : Sum  Inputs=+-
  Subtract_ff0c1 : Sum  Inputs=+-
  Blockout_d_V_f_SG_D_8_302ea : Outport
  wires:
  Divide_cd230/1 -> Subtract_f66d6/2
  State_psi_1d_SG_D_8_0200e/1 -> Product_e2d69/2
  Constant_-1_49540/1 -> Product_faebc/1
  Constant_-1_34f4d/1 -> Product_e2d69/1
  Constant_x_l_d04d7/1 -> Product_faebc/2
  Constant_x_dd_98ca9/1 -> Subtract_8f0f1/1
  State_psi_q_SG_D_8_e1efb/1 -> Product_330cc/1
  Constant_x_qdd_c31c5/1 -> Add_869b4/2
  Add_39fa3/1 -> Divide_3d3ab/2
  Subtract_ff0c1/1 -> Product_52063/2
  Constant_x_ddd_40706/1 -> Subtract_8f0f1/2
  Product_faebc/1 -> Add_869b4/1
  Constant_-1_f114f/1 -> Product_c916f/1
  State_psi_d_SG_D_8_14bfc/1 -> Product_64ce1/1
  Constant_x_l_7fa7a/1 -> Product_c916f/2
  Constant_T_A_e8e5a/1 -> Divide_26ef6/2
  Constant_x_qd_dacb6/1 -> Subtract_22882/1
  Subtract_74835/1 -> Product_f2d52/2
  Constant_x_qdd_20b45/1 -> Subtract_22882/2
  Constant_-1_d7b6c/1 -> Product_5f0f1/1
  State_psi_d_SG_D_8_c5413/1 -> Add_e38c1/2
  Constant_x_l_0f094/1 -> Product_5f0f1/2
  Constant_R_a_92b63/1 -> Product_16579/2
  Product_e2d69/1 -> Product_787ab/1
  Constant_x_qd_89036/1 -> Add_39fa3/2
  State_Px_3_SG_D_8_1b788/1 -> Product_fdd82/2
  Subtract_8f0f1/1 -> Product_787ab/2
  Constant_2.0_101c8/1 -> Product_6c9c7/1
  Constant_x_dd_b3706/1 -> Subtract_6b35b/1
  Constant_pi_70f6d/1 -> Product_6c9c7/2
  Add_e38c1/1 -> Subtract_d05d6/1
  Constant_x_l_f95df/1 -> Subtract_6b35b/2
  State_E_fd_SG_D_8_0863f/1 -> Product_2a0ae/2
  Constant_x_ddd_ec8c7/1 -> Subtract_74835/1
  Subtract_f66d6/1 -> Add_ec996/1
  Constant_x_l_4c12c/1 -> Subtract_74835/2
  State_psi_gq_SG_D_8_341db/1 -> Product_b1a5b/1
  Constant_pi_a94ab/1 -> Product_83835/2
  Add_869b4/1 -> Product_b1a5b/2
  Product_c916f/1 -> Add_39fa3/1
  Constant_x_qdd_86204/1 -> Divide_d4d57/2
  State_psi_kq_SG_D_8_85c57/1 -> Product_48e6a/1
  Subtract_22882/1 -> Product_48e6a/2
  Constant_-1_c4c0d/1 -> Product_16579/1
  Product_5f0f1/1 -> Add_a4d1c/1
  Subtract_6b35b/1 -> Divide_3899c/2
  Constant_x_qd_701ff/1 -> Add_a4d1c/2
  Product_787ab/1 -> Divide_3899c/1
  State_psi_fd_SG_D_8_8705e/1 -> Product_f2d52/1
  Constant_x_dd_cac58/1 -> Subtract_a86c3/1
  Constant_x_l_f87e3/1 -> Subtract_a86c3/2
  Product_b1a5b/1 -> Divide_3d3ab/1
  Product_48e6a/1 -> Divide_cd230/1
  State_psi_q_SG_D_8_d5d6d/1 -> Add_ec996/2
  Product_16579/1 -> Product_1b423/1
  Add_a4d1c/1 -> Divide_cd230/2
  Divide_3899c/1 -> Add_e38c1/1
  Product_f2d52/1 -> Divide_99b21/1
  Subtract_a86c3/1 -> Divide_99b21/2
  Constant_f0_e48ca/1 -> Product_53bce/2
  Divide_3d3ab/1 -> Subtract_f66d6/1
  Divide_99b21/1 -> Subtract_d05d6/2
  Constant_2.0_31101/1 -> Product_83835/1
  Subtract_d05d6/1 -> Product_1b423/2
  State_w_SG_D_8_6dc7e/1 -> Product_330cc/2
  Product_83835/1 -> Product_53bce/1
  Constant_-1_d63c0/1 -> Product_2a0ae/1
  Constant_R_a_3ed32/1 -> Product_35471/1
  Add_ec996/1 -> Product_35471/2
  State_w_SG_D_8_608f6/1 -> Product_64ce1/2
  Product_6c9c7/1 -> Product_8a692/1
  Constant_f0_ec27d/1 -> Product_8a692/2
  Product_1b423/1 -> Divide_24bb1/1
  Constant_x_ddd_32f4a/1 -> Divide_24bb1/2
  Product_330cc/1 -> Divide_55dcc/1
  Product_53bce/1 -> Divide_55dcc/2
  Product_9893f/1 -> Product_6354b/1
  Product_35471/1 -> Divide_d4d57/1
  Product_64ce1/1 -> Divide_426dd/1
  Product_8a692/1 -> Divide_426dd/2
  Divide_24bb1/1 -> Add_71666/1
  Divide_55dcc/1 -> Add_71666/2
  Product_6354b/1 -> Divide_f3605/1
  Divide_d4d57/1 -> Add_d91c7/1
  Divide_426dd/1 -> Add_d91c7/2
  Add_71666/1 -> Power_8153a/1
  Constant_2.0_848d9/1 -> Power_8153a/2
  Add_d91c7/1 -> Power_ff6be/1
  Constant_2.0_2f662/1 -> Power_ff6be/2
  Product_2a0ae/1 -> Product_9893f/1
  Constant_K_A_9f3fa/1 -> Product_9893f/2
  Constant_K_s_9d418/1 -> Product_fdd82/1
  Power_8153a/1 -> Add_e847a/1
  Power_ff6be/1 -> Add_e847a/2
  Constant_K_F_41766/1 -> Product_6354b/2
  Product_fdd82/1 -> Add_1018c/1
  Constant_V_ref_11096/1 -> Add_1018c/2
  Add_e847a/1 -> MathFunc_sqrt_98bde/1
  Constant_T_F_b010f/1 -> Divide_f3605/2
  Constant_K_A_4082f/1 -> Product_a59a3/1
  State_R_f_SG_D_8_6736f/1 -> Product_a59a3/2
  Add_1018c/1 -> Subtract_ff0c1/1
  MathFunc_sqrt_98bde/1 -> Subtract_ff0c1/2
  Divide_f3605/1 -> Add_1dd28/1
  Product_a59a3/1 -> Add_1dd28/2
  Constant_K_A_88a86/1 -> Product_52063/1
  Add_1dd28/1 -> Add_5748c/1
  Product_52063/1 -> Add_5748c/2
  Add_5748c/1 -> Subtract_bf5dd/1
  State_V_f_SG_D_8_f18fe/1 -> Subtract_bf5dd/2
  Subtract_bf5dd/1 -> Divide_26ef6/1
  Divide_26ef6/1 -> Blockout_d_V_f_SG_D_8_302ea/1

== system IEEE14_case/SG_D_8/d_psi_1d_SG_D_8_block ==
  note: d_psi_1d_SG_D_8 in case14gfl
      | $-\frac{\psi _{\mathrm{1d},\mathrm{SG},D,8}-\psi _{\mathrm{fd},\mathrm{SG},D,8}+\frac{\left(x_{\mathrm{dd}}-x_{l}\right)\,\left(\frac{\psi _{\mathrm{1d},\mathrm{SG},D,8}\,\left(x_{\mathrm{dd}}-x_{\mathrm{ddd}}\right)}{x_{\mathrm{dd}}-x_{l}}-\psi _{d,\mathrm{SG},D,8}+\frac{\psi _{\mathrm{fd},\mathrm{SG},D,8}\,\left(x_{\mathrm{ddd}}-x_{l}\right)}{x_{\mathrm{dd}}-x_{l}}\right)}{x_{\mathrm{ddd}}}}{T_{\mathrm{ddd}}}$
      | Automatically generated on 2025-10-09 21:34:01 .
  State_psi_1d_SG_D_8_961b1 : Inport
  State_psi_fd_SG_D_8_4604f : Inport  Port=2
  State_psi_1d_SG_D_8_0fd5c : Inport  Port=3
  State_psi_d_SG_D_8_df1ee : Inport  Port=4
  State_psi_fd_SG_D_8_c65e7 : Inport  Port=5
  Add_32aee : Sum
  Add_97357 : Sum
  Add_ee438 : Sum
  Constant_-1_3f196 : Constant  Value=-1
  Constant_-1_d5dba : Constant  Value=-1
  Constant_T_ddd_32816 : Constant  Value=T_ddd
  Constant_x_dd_1c9cc : Constant  Value=x_dd
  Constant_x_dd_2614a : Constant  Value=x_dd
  Constant_x_dd_411f3 : Constant  Value=x_dd
  Constant_x_dd_dde56 : Constant  Value=x_dd
  Constant_x_ddd_334c5 : Constant  Value=x_ddd
  Constant_x_ddd_50bf4 : Constant  Value=x_ddd
  Constant_x_ddd_e8d47 : Constant  Value=x_ddd
  Constant_x_l_4b417 : Constant  Value=x_l
  Constant_x_l_54690 : Constant  Value=x_l
  Constant_x_l_aded8 : Constant  Value=x_l
  Constant_x_l_f6478 : Constant  Value=x_l
  Divide_1ffdf : Product  Inputs=*/
  Divide_a927a : Product  Inputs=*/
  Divide_c16b2 : Product  Inputs=*/
  Divide_ffd6b : Product  Inputs=*/
  Product_0d74a : Product
  Product_531e3 : Product
  Product_5bc2a : Product
  Product_cd3ae : Product
  Product_f171b : Product
  Subtract_296e1 : Sum  Inputs=+-
  Subtract_39ad0 : Sum  Inputs=+-
  Subtract_4823e : Sum  Inputs=+-
  Subtract_60dcf : Sum  Inputs=+-
  Subtract_88d41 : Sum  Inputs=+-
  Subtract_d3582 : Sum  Inputs=+-
  Blockout_d_psi_1d_SG_D_8_20ff0 : Outport
  wires:
  Constant_-1_d5dba/1 -> Product_0d74a/1
  State_psi_1d_SG_D_8_0fd5c/1 -> Product_0d74a/2
  Constant_x_ddd_334c5/1 -> Subtract_60dcf/1
  Product_0d74a/1 -> Product_531e3/1
  Constant_x_dd_411f3/1 -> Subtract_39ad0/1
  Constant_x_ddd_e8d47/1 -> Subtract_39ad0/2
  Subtract_39ad0/1 -> Product_531e3/2
  Constant_T_ddd_32816/1 -> Divide_1ffdf/2
  Constant_x_dd_2614a/1 -> Subtract_d3582/1
  Constant_x_l_f6478/1 -> Subtract_4823e/2
  Constant_x_l_4b417/1 -> Subtract_d3582/2
  Constant_x_l_aded8/1 -> Subtract_60dcf/2
  Product_531e3/1 -> Divide_ffd6b/1
  Subtract_d3582/1 -> Divide_ffd6b/2
  State_psi_fd_SG_D_8_c65e7/1 -> Product_f171b/1
  Subtract_60dcf/1 -> Product_f171b/2
  Constant_x_dd_1c9cc/1 -> Subtract_296e1/1
  Constant_x_l_54690/1 -> Subtract_296e1/2
  Divide_ffd6b/1 -> Add_ee438/1
  State_psi_d_SG_D_8_df1ee/1 -> Add_ee438/2
  Product_f171b/1 -> Divide_c16b2/1
  Subtract_296e1/1 -> Divide_c16b2/2
  Divide_1ffdf/1 -> Blockout_d_psi_1d_SG_D_8_20ff0/1
  Constant_x_dd_dde56/1 -> Subtract_4823e/1
  Add_ee438/1 -> Subtract_88d41/1
  Divide_c16b2/1 -> Subtract_88d41/2
  Constant_-1_3f196/1 -> Product_5bc2a/1
  State_psi_1d_SG_D_8_961b1/1 -> Product_5bc2a/2
  Product_cd3ae/1 -> Divide_a927a/1
  Subtract_4823e/1 -> Product_cd3ae/1
  Subtract_88d41/1 -> Product_cd3ae/2
  Product_5bc2a/1 -> Add_97357/1
  State_psi_fd_SG_D_8_4604f/1 -> Add_97357/2
  Constant_x_ddd_50bf4/1 -> Divide_a927a/2
  Add_97357/1 -> Add_32aee/1
  Divide_a927a/1 -> Add_32aee/2
  Add_32aee/1 -> Divide_1ffdf/1

== system IEEE14_case/SG_D_8/d_psi_d_SG_D_8_block ==
  note: d_psi_d_SG_D_8 in case14gfl
      | $2\,\pi \,f_{0}\,\left(v_{d,\mathrm{SG},D,8}\,\sin\left(\theta _{\mathrm{SG},D,8}\right)-v_{q,\mathrm{SG},D,8}\,\cos\left(\theta _{\mathrm{SG},D,8}\right)+\frac{R_{a}\,\left(\frac{\psi _{\mathrm{1d},\mathrm{SG},D,8}\,\left(x_{\mathrm{dd}}-x_{\mathrm{ddd}}\right)}{x_{\mathrm{dd}}-x_{l}}-\psi _{d,\mathrm{SG},D,8}+\frac{\psi _{\mathrm{fd},\mathrm{SG},D,8}\,\left(x_{\mathrm{ddd}}-x_{l}\right)}{x_{\mathrm{dd}}-x_{l}}\right)}{x_{\mathrm{ddd}}}+\frac{\psi _{q,\mathrm{SG},D,8}\,w_{\mathrm{SG},D,8}}{2\,f_{0}\,\pi }\right)$
      | Automatically generated on 2025-10-09 21:33:51 .
  State_psi_1d_SG_D_8_3a1ac : Inport
  State_psi_d_SG_D_8_aedd8 : Inport  Port=2
  State_psi_fd_SG_D_8_f0d2e : Inport  Port=3
  Input_v_d_SG_D_8_41885 : Inport  Port=4
  State_theta_SG_D_8_aea71 : Inport  Port=5
  Input_v_q_SG_D_8_e5b6f : Inport  Port=6
  State_theta_SG_D_8_9f713 : Inport  Port=7
  State_psi_q_SG_D_8_b70d1 : Inport  Port=8
  State_w_SG_D_8_03911 : Inport  Port=9
  Add_27d23 : Sum
  Add_79ce7 : Sum
  Constant_-1_c5bcd : Constant  Value=-1
  Constant_-2.0_eb371 : Constant  Value=-2.0
  Constant_2.0_6409f : Constant  Value=2.0
  Constant_R_a_069b7 : Constant  Value=R_a
  Constant_f0_57f71 : Constant  Value=f0
  Constant_f0_f3100 : Constant  Value=f0
  Constant_pi_6e4d0 : Constant  Value=pi
  Constant_pi_ff92c : Constant  Value=pi
  Constant_x_dd_5bf1e : Constant  Value=x_dd
  Constant_x_dd_6d48f : Constant  Value=x_dd
  Constant_x_dd_ee75b : Constant  Value=x_dd
  Constant_x_ddd_9310a : Constant  Value=x_ddd
  Constant_x_ddd_c12ec : Constant  Value=x_ddd
  Constant_x_ddd_f9973 : Constant  Value=x_ddd
  Constant_x_l_24f3f : Constant  Value=x_l
  Constant_x_l_90812 : Constant  Value=x_l
  Constant_x_l_aadcb : Constant  Value=x_l
  Divide_17a25 : Product  Inputs=*/
  Divide_7d8e2 : Product  Inputs=*/
  Divide_c7546 : Product  Inputs=*/
  Divide_eed8e : Product  Inputs=*/
  MathFunc_cos_4b6bf : Trigonometry  Operator=cos
  MathFunc_sin_fb37c : Trigonometry
  Product_10943 : Product
  Product_493a7 : Product
  Product_55c4c : Product
  Product_66300 : Product
  Product_6835f : Product
  Product_87f31 : Product
  Product_96f3d : Product
  Product_a539b : Product
  Product_b77ad : Product
  Product_bd08d : Product
  Product_e7220 : Product
  Product_f2364 : Product
  Subtract_28314 : Sum  Inputs=+-
  Subtract_70aa0 : Sum  Inputs=+-
  Subtract_a729b : Sum  Inputs=+-
  Subtract_da3bd : Sum  Inputs=+-
  Subtract_db3d7 : Sum  Inputs=+-
  Subtract_e17f9 : Sum  Inputs=+-
  Subtract_fc155 : Sum  Inputs=+-
  Blockout_d_psi_d_SG_D_8_dc023 : Outport
  wires:
  Constant_-1_c5bcd/1 -> Product_66300/1
  Product_66300/1 -> Product_e7220/1
  Constant_x_l_90812/1 -> Subtract_a729b/2
  Constant_x_dd_6d48f/1 -> Subtract_fc155/1
  Subtract_fc155/1 -> Product_e7220/2
  State_psi_1d_SG_D_8_3a1ac/1 -> Product_66300/2
  Product_493a7/1 -> Blockout_d_psi_d_SG_D_8_dc023/1
  Subtract_da3bd/1 -> Divide_17a25/2
  Constant_x_dd_ee75b/1 -> Subtract_da3bd/1
  Constant_x_ddd_c12ec/1 -> Subtract_70aa0/1
  Constant_x_ddd_9310a/1 -> Subtract_fc155/2
  Constant_x_l_aadcb/1 -> Subtract_da3bd/2
  Constant_x_l_24f3f/1 -> Subtract_70aa0/2
  Product_e7220/1 -> Divide_17a25/1
  State_psi_fd_SG_D_8_f0d2e/1 -> Product_a539b/1
  Subtract_70aa0/1 -> Product_a539b/2
  Constant_f0_f3100/1 -> Product_87f31/2
  Constant_x_dd_5bf1e/1 -> Subtract_a729b/1
  Divide_17a25/1 -> Add_27d23/1
  Input_v_q_SG_D_8_e5b6f/1 -> Product_f2364/1
  State_psi_d_SG_D_8_aedd8/1 -> Add_27d23/2
  Product_a539b/1 -> Divide_eed8e/1
  Constant_pi_6e4d0/1 -> Product_96f3d/2
  Subtract_a729b/1 -> Divide_eed8e/2
  Add_27d23/1 -> Subtract_28314/1
  Divide_eed8e/1 -> Subtract_28314/2
  Constant_R_a_069b7/1 -> Product_6835f/1
  Subtract_28314/1 -> Product_6835f/2
  Product_87f31/1 -> Product_493a7/1
  State_theta_SG_D_8_aea71/1 -> MathFunc_sin_fb37c/1
  Product_6835f/1 -> Divide_c7546/1
  Constant_x_ddd_f9973/1 -> Divide_c7546/2
  Product_55c4c/1 -> Subtract_e17f9/2
  Input_v_d_SG_D_8_41885/1 -> Product_55c4c/1
  MathFunc_sin_fb37c/1 -> Product_55c4c/2
  MathFunc_cos_4b6bf/1 -> Product_f2364/2
  State_theta_SG_D_8_9f713/1 -> MathFunc_cos_4b6bf/1
  Product_10943/1 -> Product_bd08d/1
  Constant_2.0_6409f/1 -> Product_10943/1
  Constant_pi_ff92c/1 -> Product_10943/2
  Divide_c7546/1 -> Subtract_e17f9/1
  Product_b77ad/1 -> Divide_7d8e2/1
  State_psi_q_SG_D_8_b70d1/1 -> Product_b77ad/1
  State_w_SG_D_8_03911/1 -> Product_b77ad/2
  Constant_f0_57f71/1 -> Product_bd08d/2
  Constant_-2.0_eb371/1 -> Product_96f3d/1
  Subtract_e17f9/1 -> Add_79ce7/1
  Product_f2364/1 -> Add_79ce7/2
  Product_bd08d/1 -> Divide_7d8e2/2
  Product_96f3d/1 -> Product_87f31/1
  Add_79ce7/1 -> Subtract_db3d7/1
  Divide_7d8e2/1 -> Subtract_db3d7/2
  Subtract_db3d7/1 -> Product_493a7/2
